simulink model "closed_loop_control"  (Simulink 10.0)
settings: Solver=ode45  StartTime=0.0  StopTime=20  RelTol=1e-3  EnableMultiTasking=on
settings Model: Creator=akari  LastModifiedBy=linesLK
settings DataIOCC: LimitDataPoints=on  SignalLoggingSaveFormat=ModelDataLogs
settings OptimizationCC: ExpressionDepthLimit=2147483647
settings DebuggingCC: SolverPrmCheckMsg=warning  FcnCallInpInsideContextMsg=warning  StateNameClashWarn=warning
settings GRTTargetCC: GeneratePreprocessorConditionals=Disable all
settings ConfigComp: CovExternalEMLEnable=off

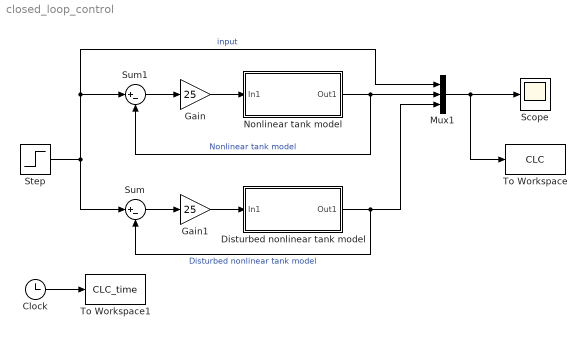
== system closed_loop_control ==
  Clock : Clock
  Disturbed nonlinear tank model : Subsystem
  Gain : Gain  Gain=25
  Gain1 : Gain  Gain=25
  Mux1 : Mux  Inputs=3
  Nonlinear tank model : Subsystem
  Scope : Scope
  Step : Step  Time=10  Before=0.6  After=1.8  SampleTime=0
  Sum : Sum  Inputs=|+-
  Sum1 : Sum  Inputs=|+-
  To Workspace : ToWorkspace  VariableName=CLC  SampleTime=-1
  To Workspace1 : ToWorkspace  VariableName=CLC_time  SampleTime=-1
  wires:
  Clock/1 -> To Workspace1/1
  Step/1 -> Sum1/1, Mux1/1, Sum/1  "input"
  Nonlinear tank model/1(Out1) -> Sum1/2, Mux1/2  "Nonlinear tank model"
  Disturbed nonlinear tank model/1(Out1) -> Sum/2, Mux1/3  "Disturbed nonlinear tank model"
  Sum1/1 -> Gain/1
  Gain/1 -> Nonlinear tank model/1(In1)
  Sum/1 -> Gain1/1
  Gain1/1 -> Disturbed nonlinear tank model/1(In1)
  Mux1/1 -> Scope/1, To Workspace/1

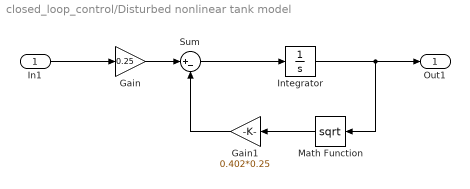
== system closed_loop_control/Disturbed nonlinear tank model ==
  In1 : Inport
  Gain : Gain  Gain=0.25
  Gain1 : Gain  Gain=0.402*0.25
  Integrator : Integrator  InitialCondition=1
  Math Function : Math  Operator=sqrt  SaturateOnIntegerOverflow=on
  Sum : Sum  Inputs=|+-
  Out1 : Outport
  wires:
  Sum/1 -> Integrator/1
  Integrator/1 -> Math Function/1, Out1/1
  Math Function/1 -> Gain1/1
  Gain/1 -> Sum/1
  Gain1/1 -> Sum/2
  In1/1 -> Gain/1

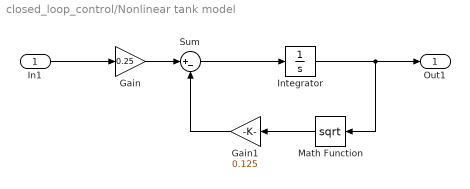
== system closed_loop_control/Nonlinear tank model ==
  In1 : Inport
  Gain : Gain  Gain=0.25
  Gain1 : Gain  Gain=0.125
  Integrator : Integrator  InitialCondition=1
  Math Function : Math  Operator=sqrt  SaturateOnIntegerOverflow=on
  Sum : Sum  Inputs=|+-
  Out1 : Outport
  wires:
  Sum/1 -> Integrator/1
  Integrator/1 -> Math Function/1, Out1/1
  Math Function/1 -> Gain1/1
  Gain/1 -> Sum/1
  Gain1/1 -> Sum/2
  In1/1 -> Gain/1
